simulink model "Progetto_Complessivo"  (R2020b)
settings: Solver=FixedStepDiscrete  StartTime=0.0  StopTime=inf  FixedStep=1/1000  RelTol=1e-3  EnableMultiTasking=on
libraries: arduinolib x5, sm_lib x4, nesl_utility x4, arduinosensorlib x2, mspfiltlib x1
settings Model: SILPILModeSetting=veronly  ExtModeTrigDuration=2  Creator=Tommaso  LastModifiedBy=Tommaso
settings OptimizationCC: EnhancedBackFolding=on  PassReuseOutputArgsAs=Individual arguments  ZeroExternalMemoryAtStartup=off  ZeroInternalMemoryAtStartup=off  MaxStackSize=64  OptimizeBlockOrder=speed  DifferentSizesBufferReuse=on  OptimizationCustomize=off  EfficientTunableParamExpr=on
settings DebuggingCC: ParameterTunabilityLossMsg=error
settings HardwareCC: ProdBitPerInt=16  ProdBitPerPointer=16  ProdBitPerSizeT=16  ProdBitPerPtrDiffT=16  ProdLargestAtomicFloat=None  ProdWordSize=8  ProdHWDeviceType=Atmel->AVR  UseEmbeddedCoderFeatures=off  UseSimulinkCoderFeatures=off
settings SFSimCC: MATLABDynamicMemAlloc=off
settings RTWCC: Description=Embedded Coder  SystemTargetFile=ert.tlc  HardwareBoard=Arduino Uno  TemplateMakefile=ert_default_tmf  Toolchain=Arduino AVR
settings CodeAppCC: ForceParamTrailComments=on  IgnoreCustomStorageClasses=off  OperatorAnnotations=on  SimulinkDataObjDesc=on  SFDataObjDesc=on  InsertBlockDesc=on
settings ERTTargetCC: SupportContinuousTime=on  SupportNonInlinedSFcns=on  SupportVariableSizeSignals=on  ExtModeStaticAllocSize=250

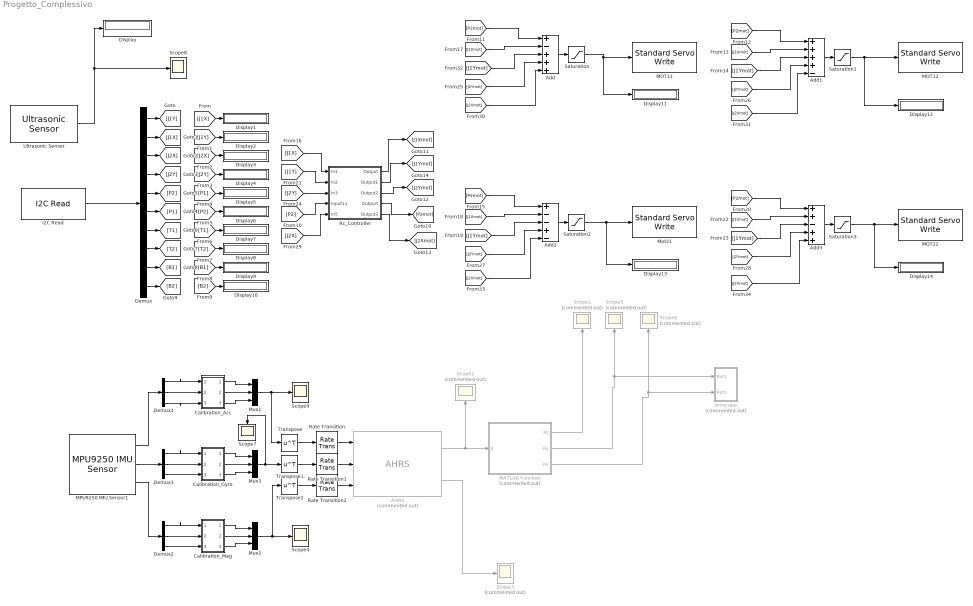
== system Progetto_Complessivo ==
  AHRS : mspfiltlib/AHRS  Commented=on  DispRefFrame=NED  DecimationFactor=1  InitialProcessNoise=ahrsfilter.defaultProcessNoise  OrientationFormat=quaternion  SimulateUsing=Code generation  AccelerometerNoise=0.05  GyroscopeNoise=1  MagnetometerNoise=3  GyroscopeDriftNoise=3.0462e-3  LinearAccelerationNoise=0.01  MagneticDisturbanceNoise=0.5  LinearAccelerationDecayFactor=0.14  MagneticDisturbanceDecayFactor=0.08  ExpectedMagneticFieldStrength=40
      settings: SourceProductBaseCode=TF,NV
  Add : Sum  Inputs=+-+++
  Add1 : Sum  Inputs=++++-
  Add2 : Sum  Inputs=+--+-
  Add3 : Sum  Inputs=++-++
  Calibration_Acc : Subsystem
  Calibration_Gyro : Subsystem
  Calibration_Mag : Subsystem
  Demux : Demux  Outputs=10
  Demux1 : Demux  Outputs=3
  Demux2 : Demux  Outputs=3
  Demux3 : Demux  Outputs=3
  Display{,1..14} (15 alike) : Display
  I2C Read : arduinolib/I2C Read  I2CModule=0  Mode=Master  SlaveAddress=08  SlaveByteOrder=BigEndian  Direction=Receiver  RegisterAddressMode=on  RegisterAddress=0  SlaveDataType=uint8  DataLength=10  NoAck=off  RepeatedStart=off  OutputStatus=off  blockPlatform=ARDUINO  SampleTime=1/500
      settings: SourceProductBaseCode=ARDUINO
  MATLAB Function : MATLAB Function  Commented=on  TreatAsAtomicUnit=on
  MOT11 : arduinolib/Standard Servo Write  pinNumber=9  ServoIndex=0  blockPlatform=ARDUINO
  MOT12 : arduinolib/Standard Servo Write  pinNumber=6  ServoIndex=1  blockPlatform=ARDUINO
  MOT22 : arduinolib/Standard Servo Write  pinNumber=3  ServoIndex=2  blockPlatform=ARDUINO
  MPU9250 IMU Sensor1 : arduinosensorlib/MPU9250 IMU Sensor  SlaveAddress=0x68  Accel=on  AngularRate=on  Ak8963Field=on  Temperature=off  Status=off  EulerAngles=off  Quat=off  AccelRange=4G  Acceldlpf=44.8 Hz  GyroRange=250 dps  Gyrodlpf=41 Hz  DmpOdr=200 Hz  SampleTime=-1
      settings: SourceProductBaseCode=ARDUINO
  Mot21 : arduinolib/Standard Servo Write  pinNumber=5  ServoIndex=3  blockPlatform=ARDUINO
  Mux1 : Mux  Inputs=3
  Mux2 : Mux  Inputs=3
  Mux3 : Mux  Inputs=3
  Rate Transition : RateTransition
  Rate Transition1 : RateTransition
  Rate Transition2 : RateTransition
  Rc_Controller : Subsystem
  Saturation{,1..3} (4 alike) : Saturate  UpperLimit=140  LowerLimit=90  LinearizeAsGain=off
  Scope{1..3,5..6} (5 alike) : Scope  Commented=on
  Scope{4,7..9} (4 alike) : Scope
  Transpose : Math  Operator=transpose  SaturateOnIntegerOverflow=on
  Transpose1 : Math  Operator=transpose  SaturateOnIntegerOverflow=on
  Transpose2 : Math  Operator=transpose  SaturateOnIntegerOverflow=on
  Ultrasonic Sensor : arduinosensorlib/Ultrasonic Sensor  NumSignalPins=2  TrigPin=12  EchoPin=13  SignalPin=3  SampleTime_=0.05  blockPlatform=ARDUINO
      settings: SourceProductBaseCode=ARDUINO
  simscape : Subsystem  Commented=on
  wires:
  I2C Read/1 -> Demux/1
  Demux/2 -> [J1X]
  Ultrasonic Sensor/1 -> Display/1, Scope8/1
  Saturation/1 -> Display11/1, MOT11/1
  Saturation1/1 -> MOT12/1, Display12/1
  Saturation2/1 -> Mot21/1, Display13/1
  Saturation3/1 -> Display14/1, MOT22/1
  Add/1 -> Saturation/1
  Add1/1 -> Saturation1/1
  Add2/1 -> Saturation2/1
  Add3/1 -> Saturation3/1
  Demux/1 -> [J1Y]
  [J1X] -> Display1/1
  [J1Y] -> Display2/1
  [J2X] -> Display3/1
  [J2Y] -> Display4/1
  [T2] -> Display8/1
  [T1] -> Display7/1
  [P1] -> Display5/1
  [P2] -> Display6/1
  [B2] -> Display10/1
  [B1] -> Display9/1
  Demux/3 -> [J2X]
  Demux/4 -> [J2Y]
  Demux/7 -> [T1]
  Demux/9 -> [B1]
  Demux/10 -> [B2]
  Demux/8 -> [T2]
  [P2mot] -> Add/1
  [J1Xmot] -> Add/2
  [J1Ymot] -> Add/3
  Demux/5 -> [P2]
  Demux/6 -> [P1]
  [P2mot] -> Add1/1
  [J1Ymot] -> Add1/3
  [J1Xmot] -> Add1/2
  [P2mot] -> Add2/1
  [J1Ymot] -> Add2/3
  [J1Xmot] -> Add2/2
  [P2mot] -> Add3/1
  [J1Ymot] -> Add3/3
  [J1Xmot] -> Add3/2
  [J2Ymot] -> Add/4
  [J2Ymot] -> Add1/4
  [J2Ymot] -> Add2/4
  [J2Ymot] -> Add3/4
  [J2Xmot] -> Add/5
  [J2Xmot] -> Add1/5
  [J2Xmot] -> Add2/5
  [J2Xmot] -> Add3/5
  [J1X] -> Rc_Controller/1(In1)
  [J1Y] -> Rc_Controller/2(In2)
  [J2Y] -> Rc_Controller/3(In3)
  [P2] -> Rc_Controller/4(Input11)
  [J2X] -> Rc_Controller/5(In5)
  Rc_Controller/1(Output) -> [J1Xmot]
  Rc_Controller/2(Output1) -> [J1Ymot]
  Rc_Controller/3(Output2) -> [J2Ymot]
  Rc_Controller/4(Outport) -> [P2mot]
  Rc_Controller/5(Output3) -> [J2Xmot]
  Mux3/1 -> Transpose1/1, Scope7/1
  Mux2/1 -> Scope4/1, Transpose2/1
  Transpose1/1 -> Rate Transition1/1
  Rate Transition1/1 -> AHRS/2
  MATLAB Function/2(Ry) -> simscape/1(Rot1), Scope5/1
  Demux2/3 -> Calibration_Mag/3(In3)
  Rate Transition2/1 -> AHRS/3
  Calibration_Acc/3(Out3) -> Mux1/3
  Demux3/3 -> Calibration_Gyro/3(In3)
  Rate Transition/1 -> AHRS/1
  AHRS/2 -> Scope3/1
  Calibration_Mag/1(Out1) -> Mux2/1
  Transpose2/1 -> Rate Transition2/1
  MPU9250 IMU Sensor1/3 -> Demux2/1
  Demux1/2 -> Calibration_Acc/2(In2)
  Transpose/1 -> Rate Transition/1
  Demux1/3 -> Calibration_Acc/3(In3)
  Mux1/1 -> Scope9/1, Transpose/1
  MPU9250 IMU Sensor1/2 -> Demux3/1
  Calibration_Acc/1(Out1) -> Mux1/1
  Calibration_Acc/2(Out2) -> Mux1/2
  Calibration_Mag/2(Out2) -> Mux2/2
  Demux2/2 -> Calibration_Mag/2(In2)
  AHRS/1 -> Scope2/1, MATLAB Function/1(q)
  Calibration_Mag/3(Out3) -> Mux2/3
  Demux3/2 -> Calibration_Gyro/2(In2)
  Demux1/1 -> Calibration_Acc/1(In1)
  MPU9250 IMU Sensor1/1 -> Demux1/1
  Demux2/1 -> Calibration_Mag/1(In1)
  Calibration_Gyro/1(Out1) -> Mux3/1
  Demux3/1 -> Calibration_Gyro/1(In1)
  Calibration_Gyro/2(Out2) -> Mux3/2
  Calibration_Gyro/3(Out3) -> Mux3/3
  MATLAB Function/1(Rz) -> Scope1/1
  MATLAB Function/3(Rx) -> simscape/2(Rot2), Scope6/1

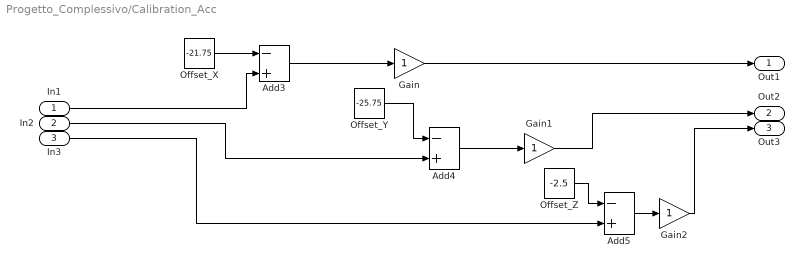
== system Progetto_Complessivo/Calibration_Acc ==
  In1 : Inport
  In2 : Inport  Port=2
  In3 : Inport  Port=3
  Add3 : Sum  Inputs=-+
  Add4 : Sum  Inputs=-+
  Add5 : Sum  Inputs=-+
  Gain : Gain
  Gain1 : Gain
  Gain2 : Gain
  Offset_X : Constant  Value=-21.75
  Offset_Y : Constant  Value=-25.75
  Offset_Z : Constant  Value=-2.5
  Out1 : Outport
  Out2 : Outport  Port=2
  Out3 : Outport  Port=3
  wires:
  Offset_Y/1 -> Add4/1
  In2/1 -> Add4/2
  Add5/1 -> Gain2/1
  Offset_X/1 -> Add3/1
  Offset_Z/1 -> Add5/1
  In3/1 -> Add5/2
  Add4/1 -> Gain1/1
  In1/1 -> Add3/2
  Add3/1 -> Gain/1
  Gain2/1 -> Out3/1
  Gain1/1 -> Out2/1
  Gain/1 -> Out1/1

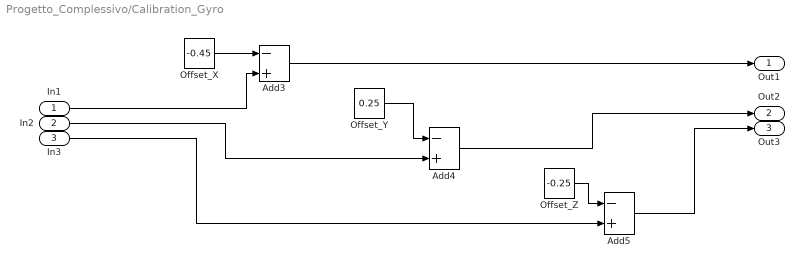
== system Progetto_Complessivo/Calibration_Gyro ==
  In1 : Inport
  In2 : Inport  Port=2
  In3 : Inport  Port=3
  Add3 : Sum  Inputs=-+
  Add4 : Sum  Inputs=-+
  Add5 : Sum  Inputs=-+
  Offset_X : Constant  Value=-0.45
  Offset_Y : Constant  Value=0.25
  Offset_Z : Constant  Value=-0.25
  Out1 : Outport
  Out2 : Outport  Port=2
  Out3 : Outport  Port=3
  wires:
  Offset_Y/1 -> Add4/1
  In2/1 -> Add4/2
  Offset_X/1 -> Add3/1
  Offset_Z/1 -> Add5/1
  In3/1 -> Add5/2
  In1/1 -> Add3/2
  Add5/1 -> Out3/1
  Add4/1 -> Out2/1
  Add3/1 -> Out1/1

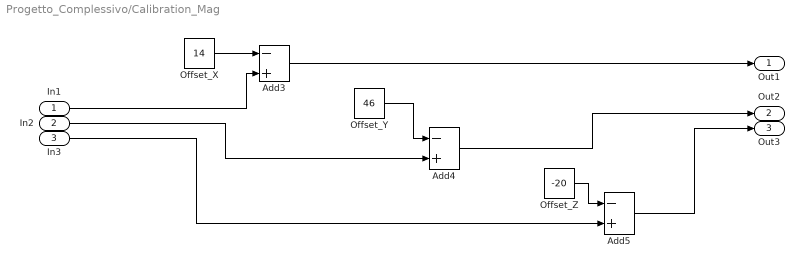
== system Progetto_Complessivo/Calibration_Mag ==
  In1 : Inport
  In2 : Inport  Port=2
  In3 : Inport  Port=3
  Add3 : Sum  Inputs=-+
  Add4 : Sum  Inputs=-+
  Add5 : Sum  Inputs=-+
  Offset_X : Constant  Value=14
  Offset_Y : Constant  Value=46
  Offset_Z : Constant  Value=-20
  Out1 : Outport
  Out2 : Outport  Port=2
  Out3 : Outport  Port=3
  wires:
  Offset_Y/1 -> Add4/1
  In2/1 -> Add4/2
  Offset_X/1 -> Add3/1
  Offset_Z/1 -> Add5/1
  In3/1 -> Add5/2
  In1/1 -> Add3/2
  Add5/1 -> Out3/1
  Add4/1 -> Out2/1
  Add3/1 -> Out1/1

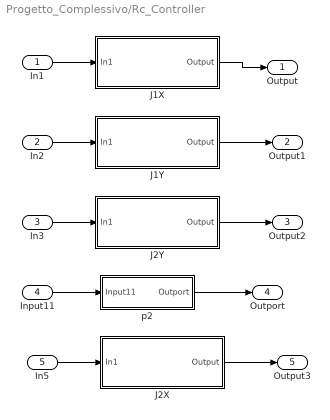
== system Progetto_Complessivo/Rc_Controller ==
  In1 : Inport
  In2 : Inport  Port=2
  In3 : Inport  Port=3
  Input11 : Inport  Port=4
  In5 : Inport  Port=5
  J1X : Subsystem
  J1Y : Subsystem
  J2X : Subsystem
  J2Y : Subsystem
  p2 : Subsystem
  Output : Outport
  Output1 : Outport  Port=2
  Output2 : Outport  Port=3
  Outport : Outport  Port=4
  Output3 : Outport  Port=5
  wires:
  Input11/1 -> p2/1(Input11)
  J2X/1(Output) -> Output3/1
  J1Y/1(Output) -> Output1/1
  In5/1 -> J2X/1(In1)
  J1X/1(Output) -> Output/1
  J2Y/1(Output) -> Output2/1
  In3/1 -> J2Y/1(In1)
  In1/1 -> J1X/1(In1)
  p2/1(Outport) -> Outport/1
  In2/1 -> J1Y/1(In1)

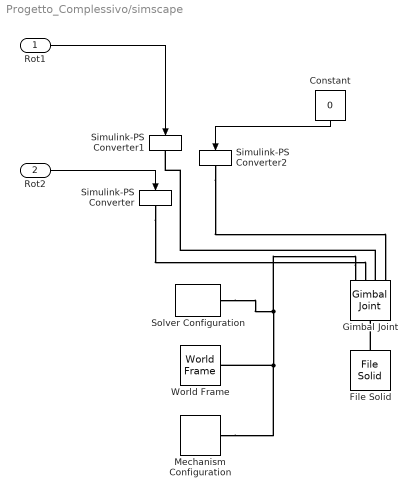
== system Progetto_Complessivo/simscape ==
  Rot1 : Inport
  Rot2 : Inport  Port=2
  Constant : Constant  Value=0
  File Solid : sm_lib/Body Elements/File Solid  ExtGeomFileName=C:\Users\Tommaso\università\Controlli Automatici\Nuovo\Relazione\GitRepo\MatlabSimulink\Ass_Global.STL  UnitType=Custom  ExtGeomFileUnits=mm  StepReaderType=HEX  ExportConvexHullGeometry=off  InertiaType=Custom  Mass=1  MassUnits=kg  CenterOfMass=[220 170 45]  CenterOfMassUnits=mm  MomentsOfInertia=[1 1 1]  MomentsOfInertiaUnits=kg*m^2  ProductsOfInertia=[0 0 0]  ProductsOfInertiaUnits=kg*m^2  BasedOnType=DensityFromFile  Density=1000  DensityUnits=kg/m^3  DoExposeReferenceFrame=off  SerializedFrames=<Frames><Frame><Id>Frame1</Id><Value><Name>F1</Name><Origin><Source>CenterOfMassFrame</Source><FeatureName></FeatureName></Origin><PrimaryAxis><DefinedDirection>+Z</DefinedDirection><Source>CenterOfMassFrame</Source><SourceDirection>+Z</SourceDirection><FeatureName></FeatureName></PrimaryAxis><SecondaryAxis><DefinedDirection>+X</DefinedDirection><Source>CenterOfMassFrame</Source><SourceDirection>+X</SourceDirection><FeatureName></FeatureName></SecondaryAxis></Value></Frame></Frames>  GraphicType=FromGeometry  MarkerShape=Sphere  MarkerSize=10  GraphicVisPropType=SimpleVisualProperties  GraphicDiffuseColor=[0.6 0.6 0.6]  GraphicSpecularColor=[0.5 0.5 0.5 1.0]  GraphicAmbientColor=[0.15 0.15 0.15 1.0]  GraphicEmissiveColor=[0.0 0.0 0.0 1.0]  GraphicShininess=75  GraphicOpacity=1.0
  Gimbal Joint : sm_lib/Joints/Gimbal Joint  JointMode=Normal  SenseConstraintForce=off  SenseConstraintForceX=off  SenseConstraintForceY=off  SenseConstraintForceZ=off  SenseConstraintTorque=off  SenseConstraintTorqueX=off  SenseConstraintTorqueY=off  SenseConstraintTorqueZ=off  SenseTotalForce=off  SenseTotalForceX=off  SenseTotalForceY=off  SenseTotalForceZ=off  SenseTotalTorque=off  SenseTotalTorqueX=off  SenseTotalTorqueY=off  SenseTotalTorqueZ=off  CompositeWrenchDir=FollowerOnBase  CompositeWrenchFrame=BaseFrame  RxEquilibriumPosition=0  RxEquilibriumPositionUnits=deg  RxSpringStiffness=0  RxSpringStiffnessUnits=N*m/deg  RxDampingCoefficient=0  RxDampingCoefficientUnits=N*m/(deg/s)  RxTorqueActuationMode=ComputedTorque  RxMotionActuationMode=InputMotion  RxSensePosition=off  RxSenseVelocity=off  RxSenseAcceleration=off  RxSenseTorqueForce=off  RxSenseLowerLimitTorqueForce=off  RxSenseUpperLimitTorqueForce=off  RxLowerLimitSpecify=off  RxLowerLimitBound=-90  RxLowerLimitBoundUnits=deg  RxLowerLimitStiffness=1e4  RxLowerLimitStiffnessUnits=N*m/deg  RxLowerLimitDamping=10  RxLowerLimitDampingUnits=N*m/(deg/s)  RxLowerLimitTransitionRegionWidth=0.1  RxLowerLimitTransitionRegionWidthUnits=deg  RxUpperLimitSpecify=off  RxUpperLimitBound=90  RxUpperLimitBoundUnits=deg  RxUpperLimitStiffness=1e4  RxUpperLimitStiffnessUnits=N*m/deg  RxUpperLimitDamping=10  RxUpperLimitDampingUnits=N*m/(deg/s)  RxUpperLimitTransitionRegionWidth=0.1  RxUpperLimitTransitionRegionWidthUnits=deg  RxPositionTargetSpecify=off  RxPositionTargetPriority=High  RxPositionTargetValue=0  RxPositionTargetValueUnits=deg  RxVelocityTargetSpecify=off  RxVelocityTargetPriority=High  RxVelocityTargetValue=0  RxVelocityTargetValueUnits=deg/s  RyEquilibriumPosition=0  RyEquilibriumPositionUnits=deg  RySpringStiffness=0  RySpringStiffnessUnits=N*m/deg  RyDampingCoefficient=0  RyDampingCoefficientUnits=N*m/(deg/s)  RyTorqueActuationMode=ComputedTorque  RyMotionActuationMode=InputMotion  RySensePosition=off  RySenseVelocity=off  RySenseAcceleration=off  RySenseTorqueForce=off  RySenseLowerLimitTorqueForce=off  RySenseUpperLimitTorqueForce=off  RyLowerLimitSpecify=off  RyLowerLimitBound=-90  RyLowerLimitBoundUnits=deg  RyLowerLimitStiffness=1e4  RyLowerLimitStiffnessUnits=N*m/deg  RyLowerLimitDamping=10  RyLowerLimitDampingUnits=N*m/(deg/s)  RyLowerLimitTransitionRegionWidth=0.1  RyLowerLimitTransitionRegionWidthUnits=deg  RyUpperLimitSpecify=off  RyUpperLimitBound=90  RyUpperLimitBoundUnits=deg  RyUpperLimitStiffness=1e4  RyUpperLimitStiffnessUnits=N*m/deg  RyUpperLimitDamping=10  RyUpperLimitDampingUnits=N*m/(deg/s)  RyUpperLimitTransitionRegionWidth=0.1  RyUpperLimitTransitionRegionWidthUnits=deg  RyPositionTargetSpecify=off  RyPositionTargetPriority=High  RyPositionTargetValue=0  RyPositionTargetValueUnits=deg  RyVelocityTargetSpecify=off  RyVelocityTargetPriority=High  RyVelocityTargetValue=0  RyVelocityTargetValueUnits=deg/s  RzEquilibriumPosition=0  RzEquilibriumPositionUnits=deg  RzSpringStiffness=0  RzSpringStiffnessUnits=N*m/deg  RzDampingCoefficient=0  RzDampingCoefficientUnits=N*m/(deg/s)  RzTorqueActuationMode=ComputedTorque  RzMotionActuationMode=InputMotion  RzSensePosition=off  RzSenseVelocity=off  RzSenseAcceleration=off  RzSenseTorqueForce=off  RzSenseLowerLimitTorqueForce=off  RzSenseUpperLimitTorqueForce=off  RzLowerLimitSpecify=off  RzLowerLimitBound=-90  RzLowerLimitBoundUnits=deg  RzLowerLimitStiffness=1e4  RzLowerLimitStiffnessUnits=N*m/deg  RzLowerLimitDamping=10  RzLowerLimitDampingUnits=N*m/(deg/s)  RzLowerLimitTransitionRegionWidth=0.1  RzLowerLimitTransitionRegionWidthUnits=deg  RzUpperLimitSpecify=off  RzUpperLimitBound=90  RzUpperLimitBoundUnits=deg  RzUpperLimitStiffness=1e4  RzUpperLimitStiffnessUnits=N*m/deg  RzUpperLimitDamping=10  RzUpperLimitDampingUnits=N*m/(deg/s)  RzUpperLimitTransitionRegionWidth=0.1  RzUpperLimitTransitionRegionWidthUnits=deg  RzPositionTargetSpecify=off  RzPositionTargetPriority=High  RzPositionTargetValue=0  RzPositionTargetValueUnits=deg  RzVelocityTargetSpecify=off  RzVelocityTargetPriority=High  RzVelocityTargetValue=0  RzVelocityTargetValueUnits=deg/s
  Mechanism Configuration : sm_lib/Utilities/Mechanism Configuration  UniformGravity=Constant  GravityVector=[0 0 -9.80665]  GravityVectorUnits=m/s^2  GravityUnits=m/s^2  LinearizationDelta=0.001  JointModeTransitionNonlinearIterations=2
  Simulink-PS Converter : nesl_utility/Simulink-PS Converter  PhysicalDomain=network_engine_domain  SubClassName=ps_input  LeftPortType=input  RightPortType=output  PseudoPeriodic=off  Frequencies=[]  NoiseDistribution=none  NoiseParameters=[]  Unit=rad  AffineConversion=off  FilteringAndDerivatives=zero  SimscapeFilterOrder=1  InputFilterTimeConstant=0.001  UdotUserProvided=0
  Simulink-PS Converter1 : nesl_utility/Simulink-PS Converter  PhysicalDomain=network_engine_domain  SubClassName=ps_input  LeftPortType=input  RightPortType=output  PseudoPeriodic=off  Frequencies=[]  NoiseDistribution=none  NoiseParameters=[]  Unit=rad  AffineConversion=off  FilteringAndDerivatives=zero  SimscapeFilterOrder=1  InputFilterTimeConstant=0.001  UdotUserProvided=0
  Simulink-PS Converter2 : nesl_utility/Simulink-PS Converter  PhysicalDomain=network_engine_domain  SubClassName=ps_input  LeftPortType=input  RightPortType=output  PseudoPeriodic=off  Frequencies=[]  NoiseDistribution=none  NoiseParameters=[]  Unit=rad  AffineConversion=off  FilteringAndDerivatives=zero  SimscapeFilterOrder=1  InputFilterTimeConstant=0.001  UdotUserProvided=0
  Solver Configuration : nesl_utility/Solver Configuration  PhysicalDomain=network_engine_domain  SubClassName=solver  LeftPortType=input  RightPortType=generic  Tones=[]  Harmonics=[]  SimulateNoise=off  Profile=off  UseLocalSampling=off  EnableSwitchedLinearOptims=on  FrequencyDomain=off  UseCCode=off  RelTol=0.001  AbsTol=1e-06  MinStep=1e-09  ToWorkspace=off  RevertToSquareIcSolve=off  NumHomotopyIterations=100  PhasorMode=off  PhasorModeNumHarmonics=1  DoDC=off  ResidualTolerance=1e-09  UseLocalSolver=off  LocalSolverChoice=NE_BACKWARD_EULER_ADVANCER  LocalSolverSampleTime=0.001  DoFixedCost=off  MaxNonlinIter=3  MaxModeIter=2  ComputeImpulses=off  ImpulseIterations=2  LinearAlgebra=auto  EquationFormulation=NE_TIME_EF  DelaysMemoryBudget=1024  AutomaticFiltering=on  FilteringTimeConstant=0.001  PartitionStorageMethod=AS_NEEDED  PartitionMemoryBudget=1024  PartitionMethod=ROBUST
  World Frame : sm_lib/Frames and Transforms/World Frame
  wires:
  Rot1/1 -> Simulink-PS Converter1/1
  Constant/1 -> Simulink-PS Converter2/1
  Rot2/1 -> Simulink-PS Converter/1
  connections:
  Gimbal Joint/LConn3 -- Simulink-PS Converter1/RConn1
  Gimbal Joint/LConn1 -- World Frame/RConn1 -- Mechanism Configuration/RConn1 -- Solver Configuration/RConn1
  File Solid/LConn1 -- Gimbal Joint/RConn1
  Simulink-PS Converter/RConn1 -- Gimbal Joint/LConn2
  Simulink-PS Converter2/RConn1 -- Gimbal Joint/LConn4

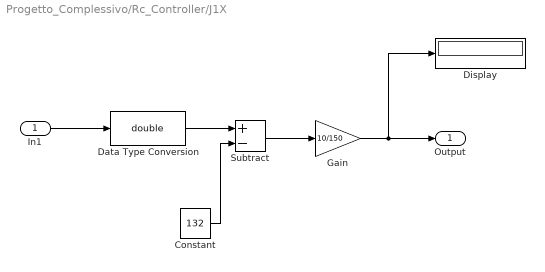
== system Progetto_Complessivo/Rc_Controller/J1X ==
  In1 : Inport
  Constant : Constant  Value=132
  Data Type Conversion : DataTypeConversion  OutDataTypeStr=double
  Display : Display
  Gain : Gain  Gain=10/150
  Subtract : Sum  Inputs=+-
  Output : Outport
  wires:
  Gain/1 -> Display/1, Output/1
  Constant/1 -> Subtract/2
  In1/1 -> Data Type Conversion/1
  Data Type Conversion/1 -> Subtract/1
  Subtract/1 -> Gain/1

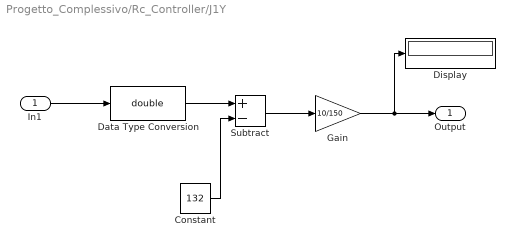
== system Progetto_Complessivo/Rc_Controller/J1Y ==
  In1 : Inport
  Constant : Constant  Value=132
  Data Type Conversion : DataTypeConversion  OutDataTypeStr=double
  Display : Display
  Gain : Gain  Gain=10/150
  Subtract : Sum  Inputs=+-
  Output : Outport
  wires:
  Gain/1 -> Display/1, Output/1
  Constant/1 -> Subtract/2
  In1/1 -> Data Type Conversion/1
  Data Type Conversion/1 -> Subtract/1
  Subtract/1 -> Gain/1

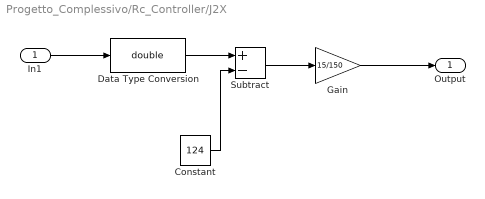
== system Progetto_Complessivo/Rc_Controller/J2X ==
  In1 : Inport
  Constant : Constant  Value=124
  Data Type Conversion : DataTypeConversion  OutDataTypeStr=double
  Gain : Gain  Gain=15/150
  Subtract : Sum  Inputs=+-
  Output : Outport
  wires:
  Gain/1 -> Output/1
  Constant/1 -> Subtract/2
  In1/1 -> Data Type Conversion/1
  Data Type Conversion/1 -> Subtract/1
  Subtract/1 -> Gain/1

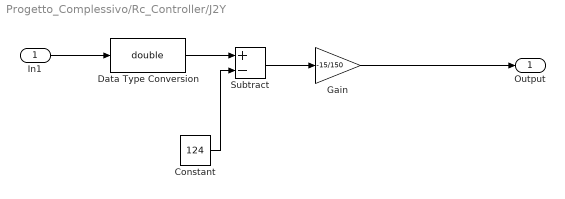
== system Progetto_Complessivo/Rc_Controller/J2Y ==
  In1 : Inport
  Constant : Constant  Value=124
  Data Type Conversion : DataTypeConversion  OutDataTypeStr=double
  Gain : Gain  Gain=-15/150
  Subtract : Sum  Inputs=+-
  Output : Outport
  wires:
  Gain/1 -> Output/1
  Constant/1 -> Subtract/2
  In1/1 -> Data Type Conversion/1
  Data Type Conversion/1 -> Subtract/1
  Subtract/1 -> Gain/1

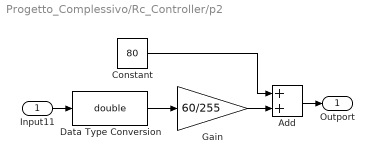
== system Progetto_Complessivo/Rc_Controller/p2 ==
  Input11 : Inport
  Add : Sum
  Constant : Constant  Value=80  OutDataTypeStr=double
  Data Type Conversion : DataTypeConversion  OutDataTypeStr=double
  Gain : Gain  Gain=60/255
  Outport : Outport
  wires:
  Gain/1 -> Add/2
  Data Type Conversion/1 -> Gain/1
  Add/1 -> Outport/1
  Constant/1 -> Add/1
  Input11/1 -> Data Type Conversion/1

== matlab function Progetto_Complessivo/MATLAB Function ==
  data: q input; Rz output; Ry output; Rx output
function [Rz, Ry, Rx] = quattoangle(q)
q0 = q(1);
q1 = q(2);
q2 = q(3);
q3 = q(4);

Rx =  atan(2*(q2*q3+q0*q1)/(q0^2-q1^2-q2^2+q3^2));
Ry =  asin(-2*(q1*q3-q0*q2));
Rz =  atan(2*(q1*q2+q0*q3)/(q0^2+q1^2-q2^2-q3^2));
end
